simulink model "Hexacopter_ControllerWithNavigation"  (R2024a)
settings: Solver=FixedStepAuto  StartTime=0.0  StopTime=inf  FixedStep=SampleTime  RelTol=1e-3  EnableMultiTasking=on
undefined symbols (not defined in the file): SampleTime
libraries: px4lib x15, slpidlib x10, px4uORBlib x7, simulink x6, uavalgslib x3, px4Sensorslib x1, simulink_extras x1, sharedutil x1, sharedtransform x1
(part 3 of 3)

== system Hexacopter_ControllerWithNavigation/Navigation/Quadcopter Navigation Algorithm/Manual Waypoints/Subsystem ==
  curr_xyzYaw : Inport
  Lookahead Point : Inport  Port=2
  Add : Sum  Inputs=+-
  Constant : Constant  Value=-1  OutDataTypeStr=Inherit: Inherit via back propagation
  Constant2 : Constant  Value=0  OutDataTypeStr=Inherit: Inherit via back propagation
  Gain : Gain
  Mux : Mux  Inputs=2
  Saturation Dynamic1 : simulink/Discontinuities/Saturation Dynamic  OutMin=0  OutMax=[]  OutDataTypeStr=Inherit: Same as second input  OutDataType=fixdt(1, 16)  OutScaling=2^-10  DoSatur=off
  Selector : Selector  InputPortWidth=4  IndexOptions=Index vector (dialog)  Indices=[3]  OutputSizes=1
  Selector1 : Selector  InputPortWidth=3  IndexOptions=Index vector (dialog)  Indices=[1 2]  OutputSizes=1
  des_landing_pos : Outport
  wires:
  Gain/1 -> Add/1
  Constant/1 -> Add/2
  Mux/1 -> des_landing_pos/1
  curr_xyzYaw/1 -> Selector/1
  Selector/1 -> Gain/1  "curr_z"
  Lookahead Point/1 -> Selector1/1
  Selector1/1 -> Mux/1  "Lookahead Point xy"
  Constant2/1 -> Saturation Dynamic1/1
  Add/1 -> Saturation Dynamic1/2, Saturation Dynamic1/3
  Saturation Dynamic1/1 -> Mux/2

== system Hexacopter_ControllerWithNavigation/Navigation/Quadcopter Navigation Algorithm/Path Correction from Onboard Computer/Define WP Yaw Values  ==
  position setpoint : Inport
  Trajectory Waypoint : Inport  Port=2
  Bus Selector : BusSelector  OutputSignals=waypoints
  Bus Selector1 : BusSelector  OutputSignals=yaw
  Bus Selector2 : BusSelector  OutputSignals=previous.yaw,next.yaw
  Data Type Conversion : DataTypeConversion  OutDataTypeStr=double  SaturateOnIntegerOverflow=off  RndMeth=Floor
  Data Type Conversion1 : DataTypeConversion  OutDataTypeStr=double  SaturateOnIntegerOverflow=off  RndMeth=Floor
  Data Type Conversion2 : DataTypeConversion  OutDataTypeStr=double  SaturateOnIntegerOverflow=off  RndMeth=Floor
  Selector : Selector  InputPortWidth=5  IndexOptions=Index vector (dialog)  Indices=1  OutputSizes=1
  Previous WP Yaw : Outport
  Current WP Yaw : Outport  Port=2
  Next WP Yaw : Outport  Port=3
  wires:
  Selector/1 -> Bus Selector1/1
  Bus Selector1/1 -> Data Type Conversion2/1  "<yaw>"
  position setpoint/1 -> Bus Selector2/1
  Bus Selector2/1 -> Data Type Conversion/1  "<yaw>"
  Bus Selector2/2 -> Data Type Conversion1/1  "<yaw>"
  Trajectory Waypoint/1 -> Bus Selector/1
  Bus Selector/1 -> Selector/1  "<waypoints>"
  Data Type Conversion/1 -> Previous WP Yaw/1
  Data Type Conversion1/1 -> Next WP Yaw/1
  Data Type Conversion2/1 -> Current WP Yaw/1

== system Hexacopter_ControllerWithNavigation/Navigation/Quadcopter Navigation Algorithm/Path Correction from Onboard Computer/Guidance Subsystem ==
  Previous WP : Inport
  Current WP : Inport  Port=2
  Next WP : Inport  Port=3
  Waypoint Type : Inport  Port=4
  Previous WP Yaw : Inport  Port=5
  Current WP Yaw : Inport  Port=6
  Next WP Yaw : Inport  Port=7
  Current Position : Inport  Port=8
  Planned_current_pos : Inport  Port=9
  planned_current_yaw : Inport  Port=10
  IDLE : Subsystem  TreatAsAtomicUnit=on
  If : If  IfExpression=(u1 ==3)  ElseIfExpressions=u1 ==4, u1 == 0
  Land : Subsystem  TreatAsAtomicUnit=on
  Merge : Merge  Inputs=4
  Take-off : Subsystem  TreatAsAtomicUnit=on
  Waypoint : Subsystem  TreatAsAtomicUnit=on
  Desired_Pose : Outport
  wires:
  Previous WP/1 -> Land/3(Previous Waypoints), Waypoint/2(Previous Waypoints)
  Current WP/1 -> Land/2(Current WP), Waypoint/3(Current Waypoints), Take-off/2(Current WP)
  Merge/1 -> Desired_Pose/1
  Next WP/1 -> Waypoint/4(Next Waypoints)
  Current Position/1 -> Land/1(Current Position), IDLE/1(Current Position), Waypoint/1(Current Position), Take-off/1(Current Position)
  Waypoint Type/1 -> If/1, Waypoint/5(Waypoint Type)
  If/1 -> Take-off/Action
  Take-off/1(x_y_z_yaw) -> Merge/1
  If/2 -> Land/Action
  Land/1(x_y_z_yaw) -> Merge/2
  Waypoint/1(x_y_z_yaw) -> Merge/3
  Previous WP Yaw/1 -> Waypoint/6(Previous WP Yaw)
  Current WP Yaw/1 -> Waypoint/7(Current WP Yaw)
  Next WP Yaw/1 -> Waypoint/8(Next WP Yaw)
  If/3 -> Waypoint/Action
  IDLE/1(x_y_z_yaw) -> Merge/4
  If/4 -> IDLE/Action
  Planned_current_pos/1 -> Waypoint/9(planned_curr_pos)
  planned_current_yaw/1 -> Waypoint/10(planned_curr_yaw)

== system Hexacopter_ControllerWithNavigation/Navigation/Quadcopter Navigation Algorithm/Path Correction from Onboard Computer/NaN Check ==
  In1 : Inport
  IsNaN : RelationalOperator  Operator=isNaN  OutDataTypeStr=boolean  RndMeth=Simplest  InputSameDT=off
  Switch : Switch  Criteria=u2 > Threshold  SaturateOnIntegerOverflow=off  InputSameDT=off
  previous safe value : Subsystem
  Out1 : Outport
  wires:
  IsNaN/1 -> Switch/2
  previous safe value/1(Out1) -> Switch/1
  Switch/1 -> Out1/1
  In1/1 -> IsNaN/1, Switch/3, previous safe value/1(In1)

== system Hexacopter_ControllerWithNavigation/Navigation/Quadcopter Navigation Algorithm/Path Correction from Onboard Computer/NaN Check1 ==
  In1 : Inport
  IsNaN : RelationalOperator  Operator=isNaN  OutDataTypeStr=boolean  RndMeth=Simplest  InputSameDT=off
  Switch : Switch  Criteria=u2 > Threshold  SaturateOnIntegerOverflow=off  InputSameDT=off
  previous safe value : Subsystem
  Out1 : Outport
  wires:
  In1/1 -> previous safe value/1(In1), Switch/3, IsNaN/1
  Switch/1 -> Out1/1
  previous safe value/1(Out1) -> Switch/1
  IsNaN/1 -> Switch/2

== system Hexacopter_ControllerWithNavigation/Navigation/Quadcopter Navigation Algorithm/Path Correction from Onboard Computer/NaN Check2 ==
  In1 : Inport
  IsNaN : RelationalOperator  Operator=isNaN  OutDataTypeStr=boolean  RndMeth=Simplest  InputSameDT=off
  Switch : Switch  Criteria=u2 > Threshold  SaturateOnIntegerOverflow=off  InputSameDT=off
  previous safe value : Subsystem
  Out1 : Outport
  wires:
  IsNaN/1 -> Switch/2
  previous safe value/1(Out1) -> Switch/1
  Switch/1 -> Out1/1
  In1/1 -> IsNaN/1, Switch/3, previous safe value/1(In1)

== system Hexacopter_ControllerWithNavigation/Navigation/Quadcopter Navigation Algorithm/Path Correction from Onboard Computer/NaN Check3 ==
  In1 : Inport
  IsNaN : RelationalOperator  Operator=isNaN  OutDataTypeStr=boolean  RndMeth=Simplest  InputSameDT=off
  Switch : Switch  Criteria=u2 > Threshold  SaturateOnIntegerOverflow=off  InputSameDT=off
  previous safe value : Subsystem
  Out1 : Outport
  wires:
  In1/1 -> previous safe value/1(In1), Switch/3, IsNaN/1
  Switch/1 -> Out1/1
  previous safe value/1(Out1) -> Switch/1
  IsNaN/1 -> Switch/2

== system Hexacopter_ControllerWithNavigation/Navigation/Quadcopter Navigation Algorithm/Path Correction from Onboard Computer/NaN Check4 ==
  In1 : Inport
  IsNaN : RelationalOperator  Operator=isNaN  OutDataTypeStr=boolean  RndMeth=Simplest  InputSameDT=off
  Switch : Switch  Criteria=u2 > Threshold  SaturateOnIntegerOverflow=off  InputSameDT=off
  previous safe value : Subsystem
  Out1 : Outport
  wires:
  IsNaN/1 -> Switch/2
  previous safe value/1(Out1) -> Switch/1
  Switch/1 -> Out1/1
  In1/1 -> IsNaN/1, Switch/3, previous safe value/1(In1)

== system Hexacopter_ControllerWithNavigation/Navigation/Quadcopter Navigation Algorithm/Path Correction from Onboard Computer/NaN Check5 ==
  In1 : Inport
  IsNaN : RelationalOperator  Operator=isNaN  OutDataTypeStr=boolean  RndMeth=Simplest  InputSameDT=off
  Switch : Switch  Criteria=u2 > Threshold  SaturateOnIntegerOverflow=off  InputSameDT=off
  previous safe value : Subsystem
  Out1 : Outport
  wires:
  In1/1 -> previous safe value/1(In1), Switch/3, IsNaN/1
  Switch/1 -> Out1/1
  previous safe value/1(Out1) -> Switch/1
  IsNaN/1 -> Switch/2

== system Hexacopter_ControllerWithNavigation/Navigation/Quadcopter Navigation Algorithm/Read waypoint from QGroundControl Mission/Guidance Subsystem ==
  Previous WP : Inport
  Current WP : Inport  Port=2
  Next WP : Inport  Port=3
  Waypoint Type : Inport  Port=4
  Current Position : Inport  Port=5
  IDLE : Subsystem  TreatAsAtomicUnit=on
  If : If  IfExpression=(u1 ==3)  ElseIfExpressions=u1 ==4, u1==0
  Land : Subsystem  TreatAsAtomicUnit=on
  Merge : Merge  Inputs=4
  Take-off : Subsystem  TreatAsAtomicUnit=on
  Waypoint : Subsystem  TreatAsAtomicUnit=on
  Desired_Pose : Outport
  wires:
  Previous WP/1 -> Land/3(Previous Waypoints), Waypoint/2(Previous Waypoints)
  Current WP/1 -> Take-off/2(Current WP), Land/2(Current WP), Waypoint/3(Current Waypoints)
  Merge/1 -> Desired_Pose/1
  Next WP/1 -> Waypoint/4(Next Waypoints)
  Current Position/1 -> Take-off/1(Current Position), Land/1(Current Position), IDLE/1(Current Position), Waypoint/1(Current Position)
  Waypoint Type/1 -> Waypoint/5(Waypoint Type), If/1
  If/1 -> Take-off/Action
  If/4 -> IDLE/Action
  Take-off/1(x_y_z_yaw) -> Merge/1
  If/2 -> Land/Action
  Land/1(x_y_z_yaw) -> Merge/2
  Waypoint/1(x_y_z_yaw) -> Merge/3
  IDLE/1(x_y_z_yaw) -> Merge/4
  If/3 -> Waypoint/Action

== system Hexacopter_ControllerWithNavigation/Navigation/Quadcopter Navigation Algorithm/Path Correction from Onboard Computer/Guidance Subsystem/IDLE ==
  Current Position : Inport
  Action Port : ActionPort  InitializeStates=reset
  Maintain Current Yaw during IDLE : Subsystem
  Mux : Mux  Inputs=2
  Reshape1 : Reshape  OutputDimensionality=Row vector (2-D)
  Selector : Selector  InputPortWidth=4  IndexOptions=Index vector (dialog)  Indices=[4]  OutputSizes=1
  Selector1 : Selector  InputPortWidth=4  IndexOptions=Index vector (dialog)  Indices=[1 2 3]  OutputSizes=1
  x_y_z_yaw : Outport
  wires:
  Maintain Current Yaw during IDLE/1(yaw_Out) -> Mux/2
  Current Position/1 -> Selector/1, Selector1/1
  Selector/1 -> Maintain Current Yaw during IDLE/1(yaw_In)
  Selector1/1 -> Mux/1
  Mux/1 -> Reshape1/1
  Reshape1/1 -> x_y_z_yaw/1

== system Hexacopter_ControllerWithNavigation/Navigation/Quadcopter Navigation Algorithm/Path Correction from Onboard Computer/Guidance Subsystem/Land ==
  Current Position : Inport
  Current WP : Inport  Port=2
  Previous Waypoints : Inport  Port=3
  Action Port : ActionPort  InitializeStates=reset
  Delay : Delay  DelayLength=1
  Ensure Smooth descend during Land : Subsystem
  IsNaN : RelationalOperator  Operator=isNaN  OutDataTypeStr=boolean  RndMeth=Simplest  InputSameDT=off
  Maintain Current Yaw during Land : Subsystem
  Mux : Mux  Inputs=3
  OR : Logic  Operator=OR  Inputs=1  IconShape=distinctive  AllPortsSameDT=off  OutDataTypeStr=boolean
  Reshape : Reshape  OutputDimensionality=Row vector (2-D)
  Reshape1 : Reshape  OutputDimensionality=Row vector (2-D)
  Selector : Selector  InputPortWidth=4  IndexOptions=Index vector (dialog)  Indices=[4]  OutputSizes=1
  Selector1 : Selector  InputPortWidth=3  IndexOptions=Index vector (dialog)  Indices=[1 2]  OutputSizes=1
  Selector2 : Selector  InputPortWidth=4  IndexOptions=Index vector (dialog)  Indices=[1 2]  OutputSizes=1
  Switch : Switch  Criteria=u2 > Threshold  SaturateOnIntegerOverflow=off  InputSameDT=off
  x_y_z_yaw : Outport
  wires:
  Maintain Current Yaw during Land/1(yaw_Out) -> Mux/3
  Selector1/1 -> Switch/3, IsNaN/1
  Ensure Smooth descend during Land/1(z) -> Mux/2
  Previous Waypoints/1 -> Ensure Smooth descend during Land/1(Previous Waypoints)
  Selector/1 -> Maintain Current Yaw during Land/1(yaw_In)
  Switch/1 -> Mux/1
  Current WP/1 -> Ensure Smooth descend during Land/2(Current WP), Selector1/1
  IsNaN/1 -> OR/1
  Selector2/1 -> Reshape1/1
  Reshape1/1 -> Delay/1
  OR/1 -> Switch/2
  Mux/1 -> Reshape/1
  Current Position/1 -> Selector2/1, Selector/1
  Reshape/1 -> x_y_z_yaw/1
  Delay/1 -> Switch/1

== system Hexacopter_ControllerWithNavigation/Navigation/Quadcopter Navigation Algorithm/Path Correction from Onboard Computer/Guidance Subsystem/Take-off ==
  Current Position : Inport
  Current WP : Inport  Port=2
  Action Port : ActionPort  InitializeStates=reset
  Demux : Demux
  Demux1 : Demux  Outputs=3
  Ensure smooth ascend during Takeoff : Subsystem
  Maintain Current Yaw during TakeOff : Subsystem
  Mux : Mux
  Reshape : Reshape  OutputDimensionality=Row vector (2-D)
  Terminator1 : Terminator
  Terminator2 : Terminator
  Terminator3 : Terminator
  x_y_z_yaw : Outport
  wires:
  Current Position/1 -> Demux/1
  Mux/1 -> Reshape/1
  Current WP/1 -> Demux1/1
  Demux/3 -> Terminator3/1
  Demux/1 -> Terminator1/1
  Demux/2 -> Terminator2/1
  Demux1/1 -> Mux/1
  Demux1/2 -> Mux/2
  Reshape/1 -> x_y_z_yaw/1
  Demux/4 -> Maintain Current Yaw during TakeOff/1(yaw_In)
  Maintain Current Yaw during TakeOff/1(yaw_Out) -> Mux/4
  Ensure smooth ascend during Takeoff/1(Out1) -> Mux/3
  Demux1/3 -> Ensure smooth ascend during Takeoff/1(In1)

== system Hexacopter_ControllerWithNavigation/Navigation/Quadcopter Navigation Algorithm/Path Correction from Onboard Computer/Guidance Subsystem/Waypoint ==
  Current Position : Inport
  Previous Waypoints : Inport  Port=2
  Current Waypoints : Inport  Port=3
  Next Waypoints : Inport  Port=4
  Waypoint Type : Inport  Port=5
  Previous WP Yaw : Inport  Port=6
  Current WP Yaw : Inport  Port=7
  Next WP Yaw : Inport  Port=8
  planned_curr_pos : Inport  Port=9
  planned_curr_yaw : Inport  Port=10
  Action Port : ActionPort  InitializeStates=reset
  Constant : Constant  Value=3
  Output signal conditioning : Subsystem
  Terminator : Terminator
  Terminator1 : Terminator
  UAV Waypoint Follower : uavalgslib/Waypoint Follower  UAVType=multirotor  StartFrom=first  TransitionRadiusSource=internal  TransitionRadius=2  MinLookaheadDistance=0.3  YawInput=on  ShowCrossTrackErrorOutput=off  ShowStatusOutput=off  SimulateUsing=Code generation
  Waypoints : Subsystem
  x_y_z_yaw : Outport
  wires:
  UAV Waypoint Follower/2 -> Terminator/1
  UAV Waypoint Follower/4 -> Terminator1/1
  Waypoints/2(Waypoint) -> UAV Waypoint Follower/2
  Previous Waypoints/1 -> Waypoints/2(previous)
  Current Waypoints/1 -> Waypoints/3(current)
  Output signal conditioning/1(xyzYaw) -> x_y_z_yaw/1
  Next Waypoints/1 -> Waypoints/4(next)
  UAV Waypoint Follower/3 -> Output signal conditioning/3(Desired Yaw)
  Waypoint Type/1 -> Output signal conditioning/4(Waypoint Type)
  Current Position/1 -> Waypoints/1(Estimated Pos), Output signal conditioning/1(Current Position)
  Previous WP Yaw/1 -> Waypoints/5(Previous WP Yaw)
  Current WP Yaw/1 -> Waypoints/6(Current WP Yaw)
  Next WP Yaw/1 -> Waypoints/7(Next WP Yaw)
  UAV Waypoint Follower/1 -> Output signal conditioning/2(LookAhead Point)
  Waypoints/1(Pose) -> UAV Waypoint Follower/1
  Constant/1 -> UAV Waypoint Follower/3
  planned_curr_pos/1 -> Waypoints/8(Inport)
  planned_curr_yaw/1 -> Waypoints/9(Inport1)

== system Hexacopter_ControllerWithNavigation/Navigation/Quadcopter Navigation Algorithm/Path Correction from Onboard Computer/NaN Check/previous safe value ==
  In1 : Inport
  Delay : Delay  DelayLength=1
  IsNaN1 : RelationalOperator  Operator=isNaN  OutDataTypeStr=boolean  RndMeth=Simplest  InputSameDT=off
  Switch1 : Switch  Criteria=u2 > Threshold  SaturateOnIntegerOverflow=off  InputSameDT=off
  Out1 : Outport
  wires:
  IsNaN1/1 -> Switch1/2
  Delay/1 -> Switch1/1
  Switch1/1 -> Delay/1, Out1/1
  In1/1 -> IsNaN1/1, Switch1/3

== system Hexacopter_ControllerWithNavigation/Navigation/Quadcopter Navigation Algorithm/Path Correction from Onboard Computer/NaN Check1/previous safe value ==
  In1 : Inport
  Delay : Delay  DelayLength=1
  IsNaN1 : RelationalOperator  Operator=isNaN  OutDataTypeStr=boolean  RndMeth=Simplest  InputSameDT=off
  Switch1 : Switch  Criteria=u2 > Threshold  SaturateOnIntegerOverflow=off  InputSameDT=off
  Out1 : Outport
  wires:
  In1/1 -> Switch1/3, IsNaN1/1
  Switch1/1 -> Out1/1, Delay/1
  Delay/1 -> Switch1/1
  IsNaN1/1 -> Switch1/2

== system Hexacopter_ControllerWithNavigation/Navigation/Quadcopter Navigation Algorithm/Path Correction from Onboard Computer/NaN Check2/previous safe value ==
  In1 : Inport
  Delay : Delay  DelayLength=1
  IsNaN1 : RelationalOperator  Operator=isNaN  OutDataTypeStr=boolean  RndMeth=Simplest  InputSameDT=off
  Switch1 : Switch  Criteria=u2 > Threshold  SaturateOnIntegerOverflow=off  InputSameDT=off
  Out1 : Outport
  wires:
  IsNaN1/1 -> Switch1/2
  Delay/1 -> Switch1/1
  Switch1/1 -> Delay/1, Out1/1
  In1/1 -> IsNaN1/1, Switch1/3

== system Hexacopter_ControllerWithNavigation/Navigation/Quadcopter Navigation Algorithm/Path Correction from Onboard Computer/NaN Check3/previous safe value ==
  In1 : Inport
  Delay : Delay  DelayLength=1
  IsNaN1 : RelationalOperator  Operator=isNaN  OutDataTypeStr=boolean  RndMeth=Simplest  InputSameDT=off
  Switch1 : Switch  Criteria=u2 > Threshold  SaturateOnIntegerOverflow=off  InputSameDT=off
  Out1 : Outport
  wires:
  In1/1 -> Switch1/3, IsNaN1/1
  Switch1/1 -> Out1/1, Delay/1
  Delay/1 -> Switch1/1
  IsNaN1/1 -> Switch1/2

== system Hexacopter_ControllerWithNavigation/Navigation/Quadcopter Navigation Algorithm/Path Correction from Onboard Computer/NaN Check4/previous safe value ==
  In1 : Inport
  Delay : Delay  DelayLength=1
  IsNaN1 : RelationalOperator  Operator=isNaN  OutDataTypeStr=boolean  RndMeth=Simplest  InputSameDT=off
  Switch1 : Switch  Criteria=u2 > Threshold  SaturateOnIntegerOverflow=off  InputSameDT=off
  Out1 : Outport
  wires:
  IsNaN1/1 -> Switch1/2
  Delay/1 -> Switch1/1
  Switch1/1 -> Delay/1, Out1/1
  In1/1 -> IsNaN1/1, Switch1/3

== system Hexacopter_ControllerWithNavigation/Navigation/Quadcopter Navigation Algorithm/Path Correction from Onboard Computer/NaN Check5/previous safe value ==
  In1 : Inport
  Delay : Delay  DelayLength=1
  IsNaN1 : RelationalOperator  Operator=isNaN  OutDataTypeStr=boolean  RndMeth=Simplest  InputSameDT=off
  Switch1 : Switch  Criteria=u2 > Threshold  SaturateOnIntegerOverflow=off  InputSameDT=off
  Out1 : Outport
  wires:
  In1/1 -> Switch1/3, IsNaN1/1
  Switch1/1 -> Out1/1, Delay/1
  Delay/1 -> Switch1/1
  IsNaN1/1 -> Switch1/2

== system Hexacopter_ControllerWithNavigation/Navigation/Quadcopter Navigation Algorithm/Read waypoint from QGroundControl Mission/Guidance Subsystem/IDLE ==
  Current Position : Inport
  Action Port : ActionPort  InitializeStates=reset  ActionPortLabel=else
  Maintain Current Yaw during IDLE : Subsystem
  Mux : Mux  Inputs=2
  Reshape1 : Reshape  OutputDimensionality=Row vector (2-D)
  Selector : Selector  InputPortWidth=4  IndexOptions=Index vector (dialog)  Indices=[4]  OutputSizes=1
  Selector1 : Selector  InputPortWidth=4  IndexOptions=Index vector (dialog)  Indices=[1 2 3]  OutputSizes=1
  x_y_z_yaw : Outport
  wires:
  Maintain Current Yaw during IDLE/1(yaw_Out) -> Mux/2
  Current Position/1 -> Selector/1, Selector1/1
  Selector/1 -> Maintain Current Yaw during IDLE/1(yaw_In)
  Selector1/1 -> Mux/1
  Mux/1 -> Reshape1/1
  Reshape1/1 -> x_y_z_yaw/1

== system Hexacopter_ControllerWithNavigation/Navigation/Quadcopter Navigation Algorithm/Read waypoint from QGroundControl Mission/Guidance Subsystem/Land ==
  Current Position : Inport
  Current WP : Inport  Port=2
  Previous Waypoints : Inport  Port=3
  Action Port : ActionPort  InitializeStates=reset  ActionPortLabel=elseif(u1 ==4)
  Delay : Delay  DelayLength=1
  Ensure Smooth descend during Land : Subsystem
  IsNaN : RelationalOperator  Operator=isNaN  OutDataTypeStr=boolean  RndMeth=Simplest  InputSameDT=off
  Maintain Current Yaw during Land : Subsystem
  Mux : Mux  Inputs=3
  OR : Logic  Operator=OR  Inputs=1  IconShape=distinctive  AllPortsSameDT=off  OutDataTypeStr=boolean
  Reshape : Reshape  OutputDimensionality=Row vector (2-D)
  Reshape1 : Reshape  OutputDimensionality=Row vector (2-D)
  Selector : Selector  InputPortWidth=4  IndexOptions=Index vector (dialog)  Indices=[4]  OutputSizes=1
  Selector1 : Selector  InputPortWidth=3  IndexOptions=Index vector (dialog)  Indices=[1 2]  OutputSizes=1
  Selector2 : Selector  InputPortWidth=4  IndexOptions=Index vector (dialog)  Indices=[1 2]  OutputSizes=1
  Switch : Switch  Criteria=u2 > Threshold  SaturateOnIntegerOverflow=off  InputSameDT=off
  x_y_z_yaw : Outport
  wires:
  Delay/1 -> Switch/1
  Reshape1/1 -> Delay/1
  OR/1 -> Switch/2
  Mux/1 -> Reshape/1
  Selector1/1 -> Switch/3, IsNaN/1
  Reshape/1 -> x_y_z_yaw/1
  Current Position/1 -> Selector2/1, Selector/1
  IsNaN/1 -> OR/1
  Selector2/1 -> Reshape1/1
  Current WP/1 -> Ensure Smooth descend during Land/2(Current WP), Selector1/1
  Ensure Smooth descend during Land/1(z) -> Mux/2
  Switch/1 -> Mux/1
  Previous Waypoints/1 -> Ensure Smooth descend during Land/1(Previous Waypoints)
  Maintain Current Yaw during Land/1(yaw_Out) -> Mux/3
  Selector/1 -> Maintain Current Yaw during Land/1(yaw_In)

== system Hexacopter_ControllerWithNavigation/Navigation/Quadcopter Navigation Algorithm/Read waypoint from QGroundControl Mission/Guidance Subsystem/Take-off ==
  Current Position : Inport
  Current WP : Inport  Port=2
  Action Port : ActionPort  InitializeStates=reset  ActionPortLabel=if((u1 ==3))
  Demux : Demux
  Demux1 : Demux  Outputs=3
  Ensure smooth ascend during Takeoff : Subsystem
  Maintain Current Yaw during TakeOff : Subsystem
  Mux : Mux
  Reshape : Reshape  OutputDimensionality=Row vector (2-D)
  Terminator1 : Terminator
  Terminator2 : Terminator
  Terminator3 : Terminator
  x_y_z_yaw : Outport
  wires:
  Current Position/1 -> Demux/1
  Mux/1 -> Reshape/1
  Current WP/1 -> Demux1/1
  Demux1/3 -> Ensure smooth ascend during Takeoff/1(In1)
  Demux/3 -> Terminator3/1
  Demux/1 -> Terminator1/1
  Demux/2 -> Terminator2/1
  Demux1/1 -> Mux/1
  Demux1/2 -> Mux/2
  Reshape/1 -> x_y_z_yaw/1
  Demux/4 -> Maintain Current Yaw during TakeOff/1(yaw_In)
  Maintain Current Yaw during TakeOff/1(yaw_Out) -> Mux/4
  Ensure smooth ascend during Takeoff/1(Out1) -> Mux/3

== system Hexacopter_ControllerWithNavigation/Navigation/Quadcopter Navigation Algorithm/Read waypoint from QGroundControl Mission/Guidance Subsystem/Waypoint ==
  Current Position : Inport
  Previous Waypoints : Inport  Port=2
  Current Waypoints : Inport  Port=3
  Next Waypoints : Inport  Port=4
  Waypoint Type : Inport  Port=5
  Action Port : ActionPort  InitializeStates=reset  ActionPortLabel=elseif( u1==0)
  Constant : Constant  Value=6
  Matrix Concatenate : Concatenate  NumInputs=3  Mode=Multidimensional array
  Output signal conditioning : Subsystem
  Reshape1 : Reshape
  Terminator : Terminator
  Terminator1 : Terminator
  UAV Waypoint Follower : uavalgslib/Waypoint Follower  UAVType=multirotor  StartFrom=first  TransitionRadiusSource=internal  TransitionRadius=2  MinLookaheadDistance=0.3  YawInput=off  ShowCrossTrackErrorOutput=off  ShowStatusOutput=off  SimulateUsing=Code generation
  x_y_z_yaw : Outport
  wires:
  Constant/1 -> UAV Waypoint Follower/3
  Matrix Concatenate/1 -> UAV Waypoint Follower/2
  UAV Waypoint Follower/2 -> Terminator/1
  Reshape1/1 -> UAV Waypoint Follower/1
  Output signal conditioning/1(xyzYaw) -> x_y_z_yaw/1
  Waypoint Type/1 -> Output signal conditioning/4(Waypoint Type)
  UAV Waypoint Follower/4 -> Terminator1/1
  UAV Waypoint Follower/1 -> Output signal conditioning/2(LookAhead Point)
  UAV Waypoint Follower/3 -> Output signal conditioning/3(Desired Yaw)
  Current Waypoints/1 -> Matrix Concatenate/2
  Current Position/1 -> Reshape1/1, Output signal conditioning/1(Current Position)
  Previous Waypoints/1 -> Matrix Concatenate/1
  Next Waypoints/1 -> Matrix Concatenate/3

== system Hexacopter_ControllerWithNavigation/Navigation/Quadcopter Navigation Algorithm/Path Correction from Onboard Computer/Guidance Subsystem/IDLE/Maintain Current Yaw during IDLE ==
  yaw_In : Inport
  Constant : Constant  Value=0
  Delay : Delay  DelayLength=1  InitialCondition=1
  Enabled Subsystem2 : Subsystem  TreatAsAtomicUnit=on
  yaw_Out : Outport
  wires:
  Delay/1 -> Enabled Subsystem2/Enable
  Constant/1 -> Delay/1
  yaw_In/1 -> Enabled Subsystem2/1(yaw_In)
  Enabled Subsystem2/1(yaw_Out) -> yaw_Out/1

== system Hexacopter_ControllerWithNavigation/Navigation/Quadcopter Navigation Algorithm/Path Correction from Onboard Computer/Guidance Subsystem/Land/Ensure Smooth descend during Land ==
  note: This ensures that the landing process is smooth by continously decrementing the altitude, instead of a sudden fall.
  note: This logic takes care of the case when Land waypoint altitude is not 0
  Previous Waypoints : Inport
  Current WP : Inport  Port=2
  Delay : Delay  DelayLength=1
  Enabled Subsystem : Subsystem  TreatAsAtomicUnit=on
  Gain : Gain  Gain=-1
  Gain1 : Gain  Gain=-1
  Gain2 : Gain  Gain=-1
  GreaterThan : RelationalOperator  Operator=>  OutDataTypeStr=boolean  RndMeth=Simplest  InputSameDT=off
  Rate of descent : Constant  Value=0.02
  Selector : Selector  InputPortWidth=3  IndexOptions=Index vector (dialog)  Indices=[3]  OutputSizes=1
  Selector1 : Selector  InputPortWidth=3  IndexOptions=Index vector (dialog)  Indices=[3]  OutputSizes=1
  Subtract : Sum  Inputs=+-
  Switch : Switch  Criteria=u2 > Threshold  SaturateOnIntegerOverflow=off  InputSameDT=off
  Switch1 : Switch  Criteria=u2 > Threshold  SaturateOnIntegerOverflow=off  InputSameDT=off
  z : Outport
  wires:
  Selector/1 -> Gain/1
  Enabled Subsystem/1(Out) -> Delay/1
  Delay/1 -> Switch/1, Switch/2
  Gain/1 -> Switch/3
  Rate of descent/1 -> Subtract/2
  Subtract/1 -> Switch1/3, GreaterThan/2, Enabled Subsystem/1(In), Enabled Subsystem/Enable
  Switch/1 -> Subtract/1
  Previous Waypoints/1 -> Selector/1
  Current WP/1 -> Selector1/1
  Selector1/1 -> Gain2/1
  Gain2/1 -> Switch1/1, GreaterThan/1
  GreaterThan/1 -> Switch1/2
  Gain1/1 -> z/1
  Switch1/1 -> Gain1/1

== system Hexacopter_ControllerWithNavigation/Navigation/Quadcopter Navigation Algorithm/Path Correction from Onboard Computer/Guidance Subsystem/Land/Maintain Current Yaw during Land ==
  yaw_In : Inport
  Constant : Constant  Value=0
  Delay : Delay  DelayLength=1  InitialCondition=1
  Enabled Subsystem2 : Subsystem  TreatAsAtomicUnit=on
  yaw_Out : Outport
  wires:
  Delay/1 -> Enabled Subsystem2/Enable
  Constant/1 -> Delay/1
  yaw_In/1 -> Enabled Subsystem2/1(yaw_In)
  Enabled Subsystem2/1(yaw_Out) -> yaw_Out/1

== system Hexacopter_ControllerWithNavigation/Navigation/Quadcopter Navigation Algorithm/Path Correction from Onboard Computer/Guidance Subsystem/Take-off/Ensure smooth ascend during Takeoff ==
  In1 : Inport
  Delay : Delay  DelayLength=1
  Gain : Gain  Gain=-1
  Gain1 : Gain  Gain=-1
  Rate : Constant  Value=0.01
  Relational Operator : RelationalOperator  Operator=<=  OutDataTypeStr=boolean  RndMeth=Simplest  InputSameDT=off
  Sum : Sum  Inputs=|++
  Switch : Switch  Criteria=u2 > Threshold  SaturateOnIntegerOverflow=off  InputSameDT=off
  Out1 : Outport
  wires:
  Rate/1 -> Sum/1
  Gain/1 -> Out1/1
  Relational Operator/1 -> Switch/2
  Switch/1 -> Gain/1
  In1/1 -> Gain1/1
  Sum/1 -> Relational Operator/2, Switch/3, Delay/1
  Gain1/1 -> Switch/1, Relational Operator/1
  Delay/1 -> Sum/2

== system Hexacopter_ControllerWithNavigation/Navigation/Quadcopter Navigation Algorithm/Path Correction from Onboard Computer/Guidance Subsystem/Take-off/Maintain Current Yaw during TakeOff ==
  yaw_In : Inport
  Constant : Constant  Value=0
  Delay : Delay  DelayLength=1  InitialCondition=1
  Enabled Subsystem2 : Subsystem  TreatAsAtomicUnit=on
  yaw_Out : Outport
  wires:
  Constant/1 -> Delay/1
  Delay/1 -> Enabled Subsystem2/Enable
  Enabled Subsystem2/1(yaw_Out) -> yaw_Out/1
  yaw_In/1 -> Enabled Subsystem2/1(yaw_In)

== system Hexacopter_ControllerWithNavigation/Navigation/Quadcopter Navigation Algorithm/Path Correction from Onboard Computer/Guidance Subsystem/Waypoint/Output signal conditioning ==
  Current Position : Inport
  LookAhead Point : Inport  Port=2
  Desired Yaw : Inport  Port=3
  Waypoint Type : Inport  Port=4
  Compare To Constant : simulink/Logic and Bit Operations/Compare To Constant  relop===  const=5  OutDataTypeStr=boolean
  Constant : Constant  Value=0  SampleTime=-1
  IsNaN : RelationalOperator  Operator=isNaN  OutDataTypeStr=boolean  RndMeth=Simplest  InputSameDT=off
  IsNaN1 : RelationalOperator  Operator=isNaN  OutDataTypeStr=boolean  RndMeth=Simplest  InputSameDT=off
  Matrix Concatenate1 : Concatenate  Mode=Multidimensional array  ConcatenateDimension=2
  OR : Logic  Operator=OR  IconShape=distinctive  AllPortsSameDT=off  OutDataTypeStr=boolean
  OR1 : Logic  Operator=OR  Inputs=1  IconShape=distinctive  AllPortsSameDT=off  OutDataTypeStr=boolean
  Reshape2 : Reshape  OutputDimensionality=Row vector (2-D)
  Reshape3 : Reshape  OutputDimensionality=Row vector (2-D)
  Switch : Switch  Criteria=u2 ~= 0  SaturateOnIntegerOverflow=off  InputSameDT=off
  Switch1 : Switch  Criteria=u2 > Threshold  SaturateOnIntegerOverflow=off  InputSameDT=off
  Transpose1 : Math  Operator=transpose
  xyzYaw : Outport
  wires:
  IsNaN1/1 -> OR1/1
  Reshape2/1 -> Matrix Concatenate1/2
  Matrix Concatenate1/1 -> Switch1/3
  OR/1 -> Switch1/2
  LookAhead Point/1 -> IsNaN1/1, Transpose1/1
  Compare To Constant/1 -> OR/2
  Transpose1/1 -> Matrix Concatenate1/1
  IsNaN/1 -> Switch/2
  Reshape3/1 -> Switch1/1
  Waypoint Type/1 -> Compare To Constant/1
  Switch1/1 -> xyzYaw/1
  Current Position/1 -> Reshape3/1
  OR1/1 -> OR/1
  Constant/1 -> Switch/1
  Switch/1 -> Reshape2/1
  Desired Yaw/1 -> Switch/3, IsNaN/1

== system Hexacopter_ControllerWithNavigation/Navigation/Quadcopter Navigation Algorithm/Path Correction from Onboard Computer/Guidance Subsystem/Waypoint/Waypoints ==
  Estimated Pos : Inport
  previous : Inport  Port=2
  current : Inport  Port=3
  next : Inport  Port=4
  Previous WP Yaw : Inport  Port=5
  Current WP Yaw : Inport  Port=6
  Next WP Yaw : Inport  Port=7
  Inport : Inport  Port=8
  Inport1 : Inport  Port=9
  Matrix Concatenate : Concatenate  NumInputs=4  Mode=Multidimensional array
  Matrix Concatenate{1..4} (4 alike) : Concatenate  Mode=Multidimensional array  ConcatenateDimension=2
  NAN check : Subsystem
  Reshape1 : Reshape
  Pose : Outport
  Waypoint : Outport  Port=2
  wires:
  next/1 -> Matrix Concatenate3/1
  Matrix Concatenate/1 -> Waypoint/1
  previous/1 -> Matrix Concatenate1/1
  Estimated Pos/1 -> Reshape1/1
  Reshape1/1 -> Pose/1
  Previous WP Yaw/1 -> NAN check/1(In1)
  Current WP Yaw/1 -> NAN check/2(In2)
  Next WP Yaw/1 -> NAN check/3(In3)
  Matrix Concatenate1/1 -> Matrix Concatenate/1
  Matrix Concatenate2/1 -> Matrix Concatenate/2
  Matrix Concatenate3/1 -> Matrix Concatenate/4
  NAN check/1(Out1) -> Matrix Concatenate1/2
  NAN check/2(Out2) -> Matrix Concatenate2/2
  NAN check/3(Out3) -> Matrix Concatenate3/2
  Matrix Concatenate4/1 -> Matrix Concatenate/3
  Inport/1 -> Matrix Concatenate4/1
  Inport1/1 -> NAN check/4(Inport1)
  NAN check/4(Out4) -> Matrix Concatenate4/2
  current/1 -> Matrix Concatenate2/1

== system Hexacopter_ControllerWithNavigation/Navigation/Quadcopter Navigation Algorithm/Read waypoint from QGroundControl Mission/Guidance Subsystem/IDLE/Maintain Current Yaw during IDLE ==
  yaw_In : Inport
  Constant : Constant  Value=0
  Delay : Delay  DelayLength=1  InitialCondition=1
  Enabled Subsystem2 : Subsystem  TreatAsAtomicUnit=on
  yaw_Out : Outport
  wires:
  Delay/1 -> Enabled Subsystem2/Enable
  Constant/1 -> Delay/1
  yaw_In/1 -> Enabled Subsystem2/1(yaw_In)
  Enabled Subsystem2/1(yaw_Out) -> yaw_Out/1

== system Hexacopter_ControllerWithNavigation/Navigation/Quadcopter Navigation Algorithm/Read waypoint from QGroundControl Mission/Guidance Subsystem/Land/Ensure Smooth descend during Land ==
  note: This ensures that the landing process is smooth by continously decrementing the altitude, instead of a sudden fall.
  note: This logic takes care of the case when Land waypoint altitude is not 0
  Previous Waypoints : Inport
  Current WP : Inport  Port=2
  Delay : Delay  DelayLength=1
  Enabled Subsystem : Subsystem  TreatAsAtomicUnit=on
  Gain : Gain  Gain=-1
  Gain1 : Gain  Gain=-1
  Gain2 : Gain  Gain=-1
  GreaterThan : RelationalOperator  Operator=>  OutDataTypeStr=boolean  RndMeth=Simplest  InputSameDT=off
  Rate of descent : Constant  Value=0.02
  Selector : Selector  InputPortWidth=3  IndexOptions=Index vector (dialog)  Indices=[3]  OutputSizes=1
  Selector1 : Selector  InputPortWidth=3  IndexOptions=Index vector (dialog)  Indices=[3]  OutputSizes=1
  Subtract : Sum  Inputs=+-
  Switch : Switch  Criteria=u2 > Threshold  SaturateOnIntegerOverflow=off  InputSameDT=off
  Switch1 : Switch  Criteria=u2 > Threshold  SaturateOnIntegerOverflow=off  InputSameDT=off
  z : Outport
  wires:
  Selector/1 -> Gain/1
  Enabled Subsystem/1(Out) -> Delay/1
  Delay/1 -> Switch/1, Switch/2
  Gain/1 -> Switch/3
  Rate of descent/1 -> Subtract/2
  Subtract/1 -> Switch1/3, GreaterThan/2, Enabled Subsystem/1(In), Enabled Subsystem/Enable
  Switch/1 -> Subtract/1
  Previous Waypoints/1 -> Selector/1
  Current WP/1 -> Selector1/1
  Selector1/1 -> Gain2/1
  Gain2/1 -> Switch1/1, GreaterThan/1
  GreaterThan/1 -> Switch1/2
  Gain1/1 -> z/1
  Switch1/1 -> Gain1/1

== system Hexacopter_ControllerWithNavigation/Navigation/Quadcopter Navigation Algorithm/Read waypoint from QGroundControl Mission/Guidance Subsystem/Land/Maintain Current Yaw during Land ==
  yaw_In : Inport
  Constant : Constant  Value=0
  Delay : Delay  DelayLength=1  InitialCondition=1
  Enabled Subsystem2 : Subsystem  TreatAsAtomicUnit=on
  yaw_Out : Outport
  wires:
  Delay/1 -> Enabled Subsystem2/Enable
  Constant/1 -> Delay/1
  yaw_In/1 -> Enabled Subsystem2/1(yaw_In)
  Enabled Subsystem2/1(yaw_Out) -> yaw_Out/1

== system Hexacopter_ControllerWithNavigation/Navigation/Quadcopter Navigation Algorithm/Read waypoint from QGroundControl Mission/Guidance Subsystem/Take-off/Ensure smooth ascend during Takeoff ==
  In1 : Inport
  Delay : Delay  DelayLength=1
  Gain : Gain  Gain=-1
  Gain1 : Gain  Gain=-1
  Rate : Constant  Value=0.01
  Relational Operator : RelationalOperator  Operator=<=  OutDataTypeStr=boolean  RndMeth=Simplest  InputSameDT=off
  Sum : Sum  Inputs=|++
  Switch : Switch  Criteria=u2 > Threshold  SaturateOnIntegerOverflow=off  InputSameDT=off
  Out1 : Outport
  wires:
  Rate/1 -> Sum/1
  Gain/1 -> Out1/1
  Relational Operator/1 -> Switch/2
  Switch/1 -> Gain/1
  In1/1 -> Gain1/1
  Sum/1 -> Relational Operator/2, Switch/3, Delay/1
  Gain1/1 -> Switch/1, Relational Operator/1
  Delay/1 -> Sum/2

== system Hexacopter_ControllerWithNavigation/Navigation/Quadcopter Navigation Algorithm/Read waypoint from QGroundControl Mission/Guidance Subsystem/Take-off/Maintain Current Yaw during TakeOff ==
  yaw_In : Inport
  Constant : Constant  Value=0
  Delay : Delay  DelayLength=1  InitialCondition=1
  Enabled Subsystem2 : Subsystem  TreatAsAtomicUnit=on
  yaw_Out : Outport
  wires:
  yaw_In/1 -> Enabled Subsystem2/1(yaw_In)
  Enabled Subsystem2/1(yaw_Out) -> yaw_Out/1
  Delay/1 -> Enabled Subsystem2/Enable
  Constant/1 -> Delay/1

== system Hexacopter_ControllerWithNavigation/Navigation/Quadcopter Navigation Algorithm/Read waypoint from QGroundControl Mission/Guidance Subsystem/Waypoint/Output signal conditioning ==
  Current Position : Inport
  LookAhead Point : Inport  Port=2
  Desired Yaw : Inport  Port=3
  Waypoint Type : Inport  Port=4
  Compare To Constant : simulink/Logic and Bit Operations/Compare To Constant  relop===  const=5  OutDataTypeStr=boolean
  Constant : Constant  Value=0  SampleTime=-1
  IsNaN : RelationalOperator  Operator=isNaN  OutDataTypeStr=boolean  RndMeth=Simplest  InputSameDT=off
  IsNaN1 : RelationalOperator  Operator=isNaN  OutDataTypeStr=boolean  RndMeth=Simplest  InputSameDT=off
  Matrix Concatenate1 : Concatenate  Mode=Multidimensional array  ConcatenateDimension=2
  OR : Logic  Operator=OR  IconShape=distinctive  AllPortsSameDT=off  OutDataTypeStr=boolean
  OR1 : Logic  Operator=OR  Inputs=1  IconShape=distinctive  AllPortsSameDT=off  OutDataTypeStr=boolean
  Reshape2 : Reshape  OutputDimensionality=Row vector (2-D)
  Reshape3 : Reshape  OutputDimensionality=Row vector (2-D)
  Switch : Switch  Criteria=u2 ~= 0  SaturateOnIntegerOverflow=off  InputSameDT=off
  Switch1 : Switch  Criteria=u2 > Threshold  SaturateOnIntegerOverflow=off  InputSameDT=off
  Transpose1 : Math  Operator=transpose
  xyzYaw : Outport
  wires:
  IsNaN1/1 -> OR1/1
  Reshape2/1 -> Matrix Concatenate1/2
  Matrix Concatenate1/1 -> Switch1/3
  OR/1 -> Switch1/2
  LookAhead Point/1 -> IsNaN1/1, Transpose1/1
  Compare To Constant/1 -> OR/2
  Transpose1/1 -> Matrix Concatenate1/1
  IsNaN/1 -> Switch/2
  Reshape3/1 -> Switch1/1
  Waypoint Type/1 -> Compare To Constant/1
  Switch1/1 -> xyzYaw/1
  Current Position/1 -> Reshape3/1
  OR1/1 -> OR/1
  Constant/1 -> Switch/1
  Switch/1 -> Reshape2/1
  Desired Yaw/1 -> Switch/3, IsNaN/1

== system Hexacopter_ControllerWithNavigation/Navigation/Quadcopter Navigation Algorithm/Path Correction from Onboard Computer/Guidance Subsystem/IDLE/Maintain Current Yaw during IDLE/Enabled Subsystem2 ==
  yaw_In : Inport
  Enable : EnablePort
  yaw_Out : Outport
  wires:
  yaw_In/1 -> yaw_Out/1

== system Hexacopter_ControllerWithNavigation/Navigation/Quadcopter Navigation Algorithm/Path Correction from Onboard Computer/Guidance Subsystem/Land/Ensure Smooth descend during Land/Enabled Subsystem ==
  In : Inport
  Enable : EnablePort
  Out : Outport
  wires:
  In/1 -> Out/1

== system Hexacopter_ControllerWithNavigation/Navigation/Quadcopter Navigation Algorithm/Path Correction from Onboard Computer/Guidance Subsystem/Land/Maintain Current Yaw during Land/Enabled Subsystem2 ==
  yaw_In : Inport
  Enable : EnablePort
  yaw_Out : Outport
  wires:
  yaw_In/1 -> yaw_Out/1

== system Hexacopter_ControllerWithNavigation/Navigation/Quadcopter Navigation Algorithm/Path Correction from Onboard Computer/Guidance Subsystem/Take-off/Maintain Current Yaw during TakeOff/Enabled Subsystem2 ==
  yaw_In : Inport
  Enable : EnablePort
  yaw_Out : Outport
  wires:
  yaw_In/1 -> yaw_Out/1

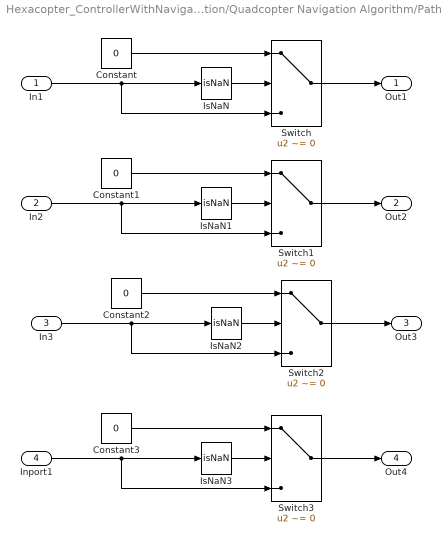
== system Hexacopter_ControllerWithNavigation/Navigation/Quadcopter Navigation Algorithm/Path Correction from Onboard Computer/Guidance Subsystem/Waypoint/Waypoints/NAN check ==
  In1 : Inport
  In2 : Inport  Port=2
  In3 : Inport  Port=3
  Inport1 : Inport  Port=4
  Constant{,1..3} (4 alike) : Constant  Value=0  SampleTime=-1
  IsNaN{,1..3} (4 alike) : RelationalOperator  Operator=isNaN  OutDataTypeStr=boolean  RndMeth=Simplest  InputSameDT=off
  Switch{,1..3} (4 alike) : Switch  Criteria=u2 ~= 0  SaturateOnIntegerOverflow=off  InputSameDT=off
  Out1 : Outport
  Out2 : Outport  Port=2
  Out3 : Outport  Port=3
  Out4 : Outport  Port=4
  wires:
  Switch/1 -> Out1/1
  In1/1 -> Switch/3, IsNaN/1
  Constant/1 -> Switch/1
  IsNaN/1 -> Switch/2
  Switch1/1 -> Out2/1
  IsNaN1/1 -> Switch1/2
  In2/1 -> Switch1/3, IsNaN1/1
  Constant1/1 -> Switch1/1
  Switch2/1 -> Out3/1
  IsNaN2/1 -> Switch2/2
  In3/1 -> Switch2/3, IsNaN2/1
  Constant2/1 -> Switch2/1
  Inport1/1 -> Switch3/3, IsNaN3/1
  Switch3/1 -> Out4/1
  Constant3/1 -> Switch3/1
  IsNaN3/1 -> Switch3/2

== system Hexacopter_ControllerWithNavigation/Navigation/Quadcopter Navigation Algorithm/Read waypoint from QGroundControl Mission/Guidance Subsystem/IDLE/Maintain Current Yaw during IDLE/Enabled Subsystem2 ==
  yaw_In : Inport
  Enable : EnablePort
  yaw_Out : Outport
  wires:
  yaw_In/1 -> yaw_Out/1

== system Hexacopter_ControllerWithNavigation/Navigation/Quadcopter Navigation Algorithm/Read waypoint from QGroundControl Mission/Guidance Subsystem/Land/Ensure Smooth descend during Land/Enabled Subsystem ==
  In : Inport
  Enable : EnablePort
  Out : Outport
  wires:
  In/1 -> Out/1

== system Hexacopter_ControllerWithNavigation/Navigation/Quadcopter Navigation Algorithm/Read waypoint from QGroundControl Mission/Guidance Subsystem/Land/Maintain Current Yaw during Land/Enabled Subsystem2 ==
  yaw_In : Inport
  Enable : EnablePort
  yaw_Out : Outport
  wires:
  yaw_In/1 -> yaw_Out/1

== system Hexacopter_ControllerWithNavigation/Navigation/Quadcopter Navigation Algorithm/Read waypoint from QGroundControl Mission/Guidance Subsystem/Take-off/Maintain Current Yaw during TakeOff/Enabled Subsystem2 ==
  yaw_In : Inport
  Enable : EnablePort
  yaw_Out : Outport
  wires:
  yaw_In/1 -> yaw_Out/1

== stateflow chart Hexacopter_ControllerWithNavigation/Position & Rate Controller/Chart ==
  state STABLIZED
    des_yawrate = RC_yawrate;
    des_pitch = RC_pitch;
    des_roll = RC_roll;
    des_thrust = RC_thrust;
  state MISSION
    des_yawrate = CTRL_yawrate;
    des_pitch = CTRL_pitch;
    des_roll = CTRL_roll;
    des_thrust = CTRL_thrust;
  (default) -> STABLIZED
  STABLIZED -> MISSION : [RC_MODE > 1400]
  MISSION -> STABLIZED : [RC_MODE <= 1400]
  data: des_pitch output; des_roll output; des_thrust output; des_yawrate output; RC_pitch input; RC_roll input; RC_thrust input; RC_yawrate input; CTRL_pitch input; CTRL_thrust input; CTRL_roll input; CTRL_yawrate input; RC_MODE input
